simulink model "zad62pendulum_22a"  (R2022a)
settings: Solver=ode4  StartTime=0.0  StopTime=25  FixedStep=0.001  RelTol=1e-3
values from neighbouring files (symbols this model uses):
  A = [0 1;g/l -c/(l*m)]    [zad62_pendulum_Main.m]
  B = [0; 1/m]    [zad62_pendulum_Main.m]
  C = [1 0]    [zad62_pendulum_Main.m]
  K = lqr(A,B,Q,R)    [zad62_pendulum_Main.m]
  Ki = zeta(2)    [zad62_pendulum_Main.m]
  Kp = Kp_set(i)    [zad61_Main.m]    (also in zad62_pendulum_Main.m = zeta(1))
  N_bar = N_xu(end)+K*N_xu(1:(end-1))    [zad62_pendulum_Main.m]
  Q = eye(2)    [zad62_pendulum_Main.m]
  R = 1    [zad62_pendulum_Main.m]
  x0 = [0.1; 0]    [zad62_pendulum_Main.m]
settings Model: Creator=henry  LastModifiedBy=henry
settings ModelReferenceCC: EnableRefExpFcnMdlSchedulingChecks=off
settings RTWCC: Description=Generic Real-Time Target

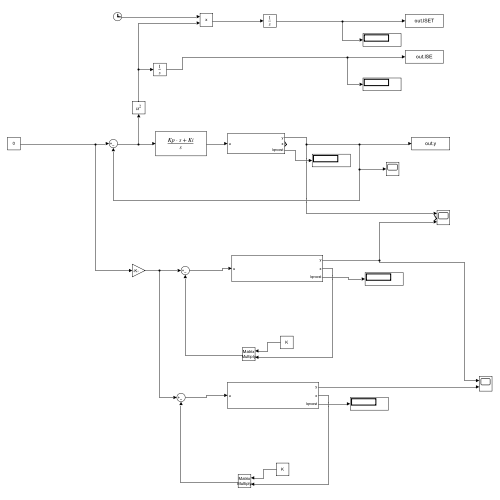
[thumbnail: Simulink's stored preview of the top-level diagram]
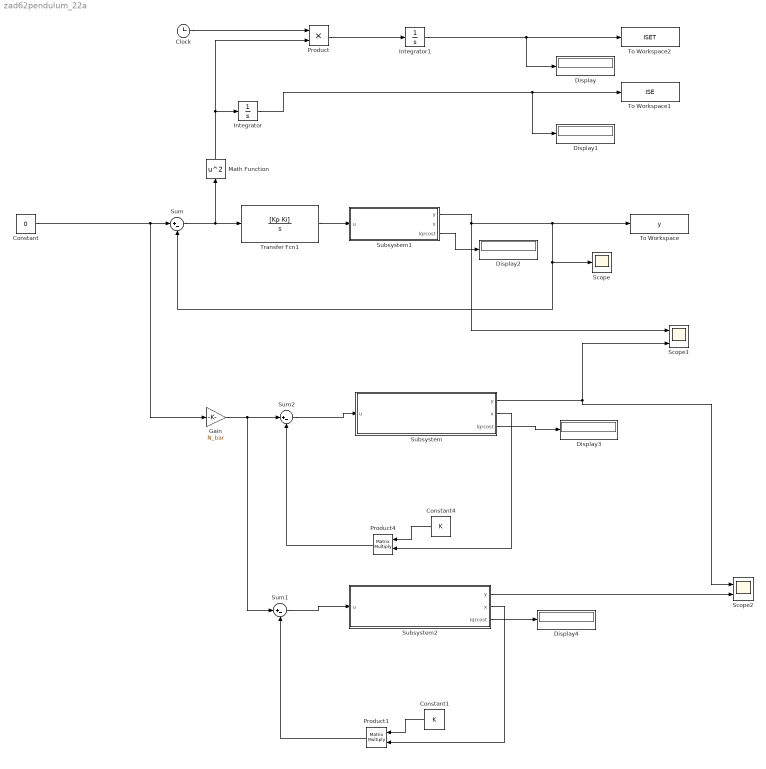
== system zad62pendulum_22a ==
  Clock : Clock
  Constant : Constant  Value=0
  Constant1 : Constant  Value=K  VectorParams1D=off
  Constant4 : Constant  Value=K  VectorParams1D=off
  Display{,1..4} (5 alike) : Display
  Gain : Gain  Gain=N_bar
  Integrator : Integrator
  Integrator1 : Integrator
  Math Function : Math  Operator=square
  Product : Product
  Product1 : Product  Multiplication=Matrix(*)
  Product4 : Product  Multiplication=Matrix(*)
  Scope : Scope
  Scope1 : Scope  NumInputPorts=3
  Scope2 : Scope  NumInputPorts=2
  Subsystem : Subsystem
  Subsystem1 : Subsystem
  Subsystem2 : Subsystem
  Sum : Sum  Inputs=|+-
  Sum1 : Sum  Inputs=|+-
  Sum2 : Sum  Inputs=|+-
  To Workspace : ToWorkspace  VariableName=y  SampleTime=-1
  To Workspace1 : ToWorkspace  VariableName=ISE  SampleTime=-1
  To Workspace2 : ToWorkspace  VariableName=ISET  SampleTime=-1
  Transfer Fcn1 : TransferFcn  Numerator=[Kp Ki]  Denominator=[1 0]
  wires:
  Transfer Fcn1/1 -> Subsystem1/1(u)
  Constant/1 -> Gain/1, Sum/1
  Sum/1 -> Transfer Fcn1/1, Math Function/1
  Subsystem1/1(y) -> Scope1/1, Scope/1, Sum/2, To Workspace/1
  Integrator/1 -> Display1/1, To Workspace1/1
  Math Function/1 -> Product/2, Integrator/1
  Product/1 -> Integrator1/1
  Integrator1/1 -> Display/1, To Workspace2/1
  Clock/1 -> Product/1
  Constant4/1 -> Product4/1
  Product4/1 -> Sum2/2
  Sum2/1 -> Subsystem/1(u)
  Subsystem/1(y) -> Scope1/3, Scope2/1
  Subsystem/2(x) -> Product4/2
  Subsystem1/3(lqrcost) -> Display2/1
  Subsystem/3(lqrcost) -> Display3/1
  Subsystem2/2(x) -> Product1/2
  Subsystem2/1(y) -> Scope2/2
  Gain/1 -> Sum1/1, Sum2/1
  Product1/1 -> Sum1/2
  Constant1/1 -> Product1/1
  Sum1/1 -> Subsystem2/1(u)
  Subsystem2/3(lqrcost) -> Display4/1

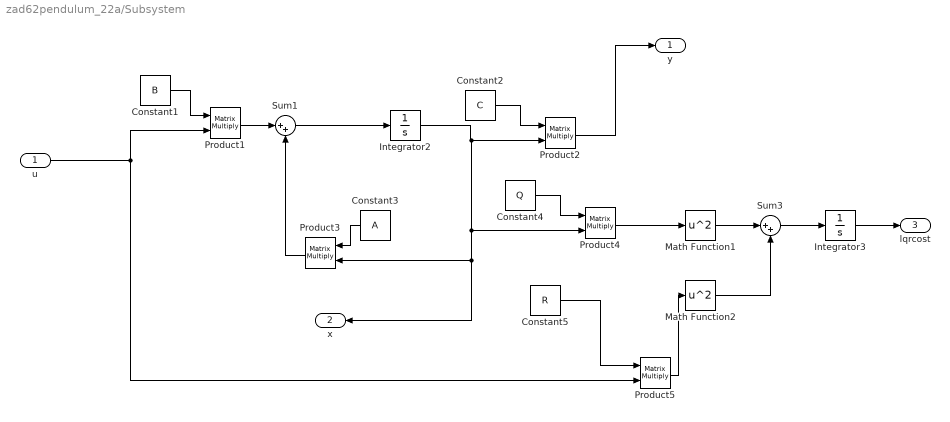
== system zad62pendulum_22a/Subsystem ==
  u : Inport
  Constant1 : Constant  Value=B
  Constant2 : Constant  Value=C  VectorParams1D=off
  Constant3 : Constant  Value=A
  Constant4 : Constant  Value=Q  VectorParams1D=off
  Constant5 : Constant  Value=R  VectorParams1D=off
  Integrator2 : Integrator  InitialCondition=x0
  Integrator3 : Integrator
  Math Function1 : Math  Operator=square
  Math Function2 : Math  Operator=square
  Product{1..5} (5 alike) : Product  Multiplication=Matrix(*)
  Sum1 : Sum  Inputs=|++
  Sum3 : Sum  Inputs=|++
  y : Outport
  x : Outport  Port=2
  lqrcost : Outport  Port=3
  wires:
  Product1/1 -> Sum1/1
  Constant2/1 -> Product2/1
  Sum1/1 -> Integrator2/1
  Constant3/1 -> Product3/1
  Product3/1 -> Sum1/2
  Constant1/1 -> Product1/1
  Integrator2/1 -> Product4/2, x/1, Product3/2, Product2/2
  u/1 -> Product5/2, Product1/2
  Product2/1 -> y/1
  Math Function2/1 -> Sum3/2
  Math Function1/1 -> Sum3/1
  Sum3/1 -> Integrator3/1
  Constant4/1 -> Product4/1
  Product4/1 -> Math Function1/1
  Constant5/1 -> Product5/1
  Product5/1 -> Math Function2/1
  Integrator3/1 -> lqrcost/1

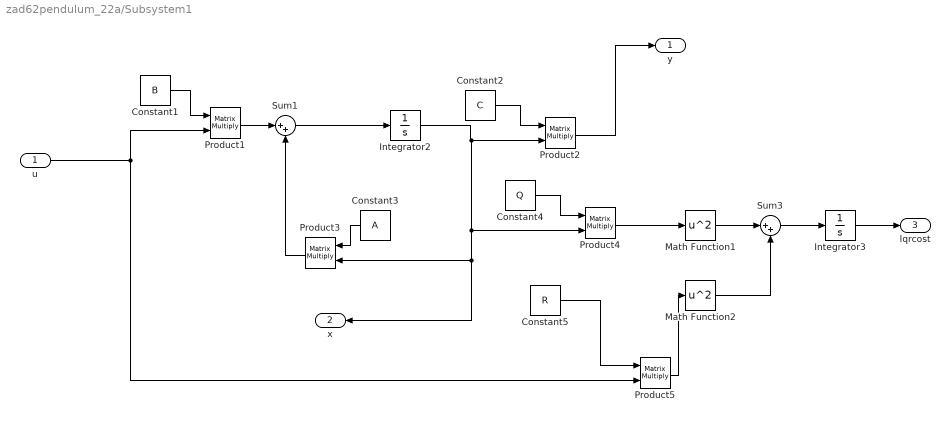
== system zad62pendulum_22a/Subsystem1 ==
  u : Inport
  Constant1 : Constant  Value=B
  Constant2 : Constant  Value=C  VectorParams1D=off
  Constant3 : Constant  Value=A
  Constant4 : Constant  Value=Q  VectorParams1D=off
  Constant5 : Constant  Value=R  VectorParams1D=off
  Integrator2 : Integrator  InitialCondition=x0
  Integrator3 : Integrator
  Math Function1 : Math  Operator=square
  Math Function2 : Math  Operator=square
  Product{1..5} (5 alike) : Product  Multiplication=Matrix(*)
  Sum1 : Sum  Inputs=|++
  Sum3 : Sum  Inputs=|++
  y : Outport
  x : Outport  Port=2
  lqrcost : Outport  Port=3
  wires:
  Integrator3/1 -> lqrcost/1
  Product5/1 -> Math Function2/1
  Constant5/1 -> Product5/1
  Product4/1 -> Math Function1/1
  Constant4/1 -> Product4/1
  Sum3/1 -> Integrator3/1
  Math Function1/1 -> Sum3/1
  Math Function2/1 -> Sum3/2
  Product2/1 -> y/1
  u/1 -> Product1/2, Product5/2
  Integrator2/1 -> Product2/2, Product3/2, x/1, Product4/2
  Constant1/1 -> Product1/1
  Product3/1 -> Sum1/2
  Constant3/1 -> Product3/1
  Sum1/1 -> Integrator2/1
  Constant2/1 -> Product2/1
  Product1/1 -> Sum1/1

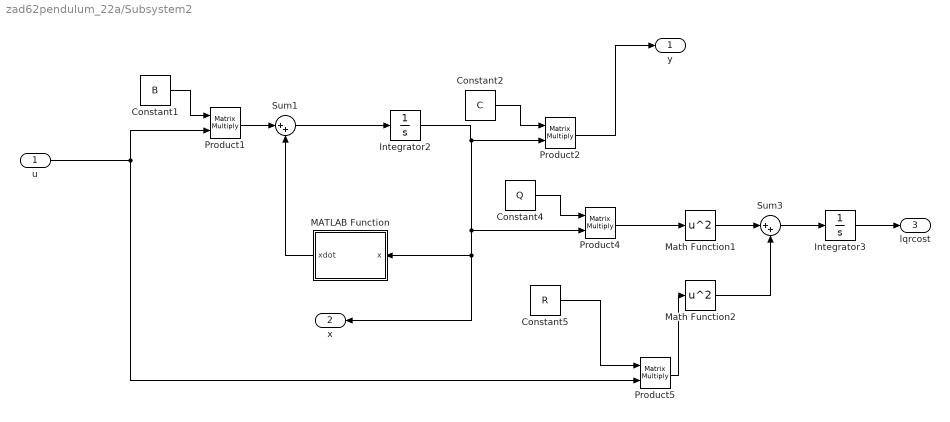
== system zad62pendulum_22a/Subsystem2 ==
  u : Inport
  Constant1 : Constant  Value=B
  Constant2 : Constant  Value=C  VectorParams1D=off
  Constant4 : Constant  Value=Q  VectorParams1D=off
  Constant5 : Constant  Value=R  VectorParams1D=off
  Integrator2 : Integrator  InitialCondition=x0
  Integrator3 : Integrator
  MATLAB Function : MATLAB Function  TreatAsAtomicUnit=on
  Math Function1 : Math  Operator=square
  Math Function2 : Math  Operator=square
  Product{1..2,4..5} (4 alike) : Product  Multiplication=Matrix(*)
  Sum1 : Sum  Inputs=|++
  Sum3 : Sum  Inputs=|++
  y : Outport
  x : Outport  Port=2
  lqrcost : Outport  Port=3
  wires:
  Integrator3/1 -> lqrcost/1
  Product5/1 -> Math Function2/1
  Constant5/1 -> Product5/1
  Product4/1 -> Math Function1/1
  Constant4/1 -> Product4/1
  Sum3/1 -> Integrator3/1
  Math Function1/1 -> Sum3/1
  Math Function2/1 -> Sum3/2
  Product2/1 -> y/1
  u/1 -> Product1/2, Product5/2
  Integrator2/1 -> Product2/2, MATLAB Function/1(x), x/1, Product4/2
  Constant1/1 -> Product1/1
  MATLAB Function/1(xdot) -> Sum1/2
  Sum1/1 -> Integrator2/1
  Constant2/1 -> Product2/1
  Product1/1 -> Sum1/1

== matlab function zad62pendulum_22a/Subsystem2/MATLAB Function ==
  data: x input; xdot output
function xdot = fcn(x)

g = 9.81;
c = 2.5;
l = 5;
m = 5;

xdot = [x(2); g/l*sin(x(1))-c/(l*m)*x(2)];
